simulink model "ISO2631_All_Generation"  (Simulink 7.6)
settings: Solver=ode45  StartTime=0.0  StopTime=1  RelTol=1e-3
settings Model: Creator=Kristian  LastModifiedBy=Kristian
settings RTWCC: GenerateReport=on  LaunchReport=on
settings SimEventsCC: propDiagAttribOutput=1  propDiagFcnCallOutput=1  propDiagStatOutput=0

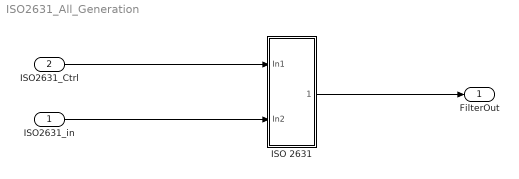
== system ISO2631_All_Generation ==
  ISO2631_in : Inport  OutDataTypeStr=double
  ISO2631_Ctrl : Inport  Port=2  OutDataTypeStr=double
  ISO 2631 : Subsystem
  FilterOut : Outport  OutDataTypeStr=double
  wires:
  ISO2631_Ctrl/1 -> ISO 2631/1(In1)
  ISO 2631/1(Out1) -> FilterOut/1
  ISO2631_in/1 -> ISO 2631/2(In2)

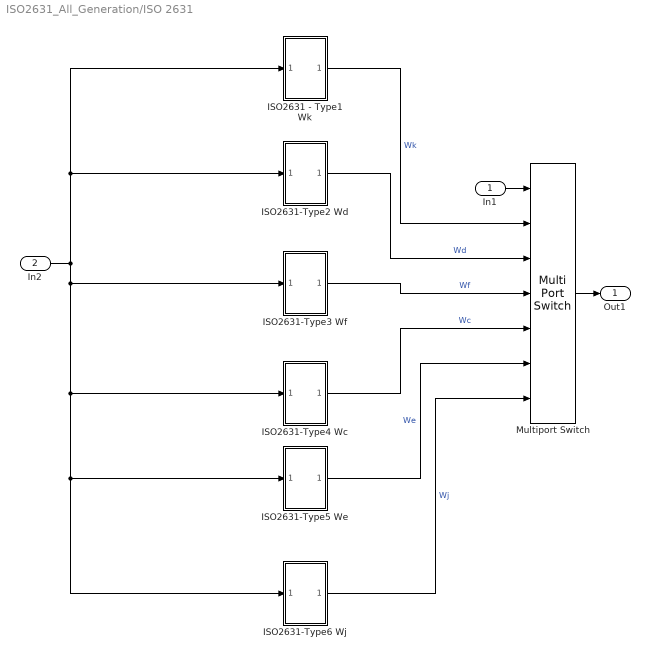
== system ISO2631_All_Generation/ISO 2631 ==
  In1 : Inport
  In2 : Inport  Port=2
  ISO2631 - Type1 Wk : Subsystem
  ISO2631-Type2 Wd : Subsystem
  ISO2631-Type3 Wf : Subsystem
  ISO2631-Type4 Wc : Subsystem
  ISO2631-Type5 We : Subsystem
  ISO2631-Type6 Wj : Subsystem
  Multiport Switch : MultiPortSwitch  DataPortOrder=Specify indices  Inputs=6  DataPortIndices={1,2,3,4,5,6}  zeroidx=off  RndMeth=Ceiling
  Out1 : Outport
  wires:
  In2/1 -> ISO2631 - Type1 Wk/1(In1), ISO2631-Type2 Wd/1(In1), ISO2631-Type3 Wf/1(In1), ISO2631-Type4 Wc/1(In1), ISO2631-Type6 Wj/1(In1), ISO2631-Type5 We/1(In1)
  ISO2631 - Type1 Wk/1(Out1) -> Multiport Switch/2  "Wk"
  ISO2631-Type2 Wd/1(Out1) -> Multiport Switch/3  "Wd"
  ISO2631-Type3 Wf/1(Out1) -> Multiport Switch/4  "Wf"
  ISO2631-Type4 Wc/1(Out1) -> Multiport Switch/5  "Wc"
  ISO2631-Type5 We/1(Out1) -> Multiport Switch/6  "We"
  ISO2631-Type6 Wj/1(Out1) -> Multiport Switch/7  "Wj"
  In1/1 -> Multiport Switch/1
  Multiport Switch/1 -> Out1/1

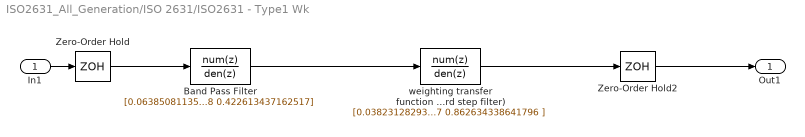
== system ISO2631_All_Generation/ISO 2631/ISO2631 - Type1 Wk ==
  In1 : Inport
  Band Pass Filter : DiscreteFilter  Numerator=|  Denominator=[1.0 -3.16470636644551 3.75293919582273 -2.01084465327318 0.422613437162517]  SampleTime=1/1000
      | [0.0638508113542868 1.33226762955019E-15 -0.127701622708578 4.2188474935756E-15 0.0638508113542855
      | ]
  Zero-Order Hold : ZeroOrderHold  SampleTime=1/1000
  Zero-Order Hold2 : ZeroOrderHold  SampleTime=1/1000
  weighting transfer function (Acceleration-velocity transition + Upward step filter) : DiscreteFilter  Numerator=|  Denominator=|  SampleTime=1/1000
      Numerator=|
      | [0.0382312829345277 -0.0729444373075823 -0.0034621921267961 0.0729450727468253 -0.0347684553684901
      | ]
      Denominator=|
      | [1.0 -3.85371908982878 5.57025894073329 -3.57917165034607 0.862634338641796
      | ]
  Out1 : Outport
  wires:
  Band Pass Filter/1 -> weighting transfer function (Acceleration-velocity transition + Upward step filter)/1
  Zero-Order Hold/1 -> Band Pass Filter/1
  In1/1 -> Zero-Order Hold/1
  weighting transfer function (Acceleration-velocity transition + Upward step filter)/1 -> Zero-Order Hold2/1
  Zero-Order Hold2/1 -> Out1/1

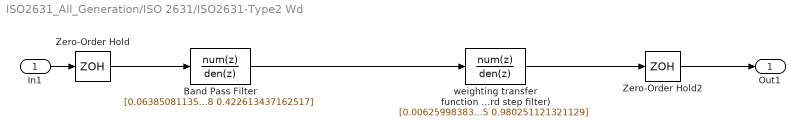
== system ISO2631_All_Generation/ISO 2631/ISO2631-Type2 Wd ==
  In1 : Inport
  Band Pass Filter : DiscreteFilter  Numerator=[0.0638508113542868 1.33226762955019e-15 -0.127701622708578 4.21884749357560e-15 0.0638508113542855]  Denominator=[1 -3.16470636644551 3.75293919582273 -2.01084465327318 0.422613437162517]  SampleTime=1/1000
  Zero-Order Hold : ZeroOrderHold  SampleTime=1/1000
  Zero-Order Hold2 : ZeroOrderHold  SampleTime=1/1000
  weighting transfer function (Acceleration-velocity transition + Upward step filter) : DiscreteFilter  Numerator=[0.00625998383111404 7.81740945390297e-05 -0.00618180973657412]  Denominator=[1 -1.98009477313205 0.980251121321129]  SampleTime=1/1000
  Out1 : Outport
  wires:
  Band Pass Filter/1 -> weighting transfer function (Acceleration-velocity transition + Upward step filter)/1
  Zero-Order Hold/1 -> Band Pass Filter/1
  In1/1 -> Zero-Order Hold/1
  weighting transfer function (Acceleration-velocity transition + Upward step filter)/1 -> Zero-Order Hold2/1
  Zero-Order Hold2/1 -> Out1/1

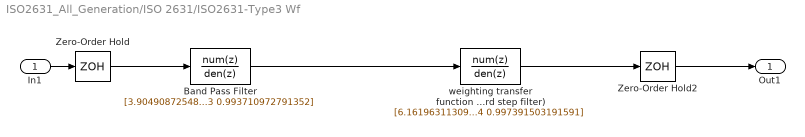
== system ISO2631_All_Generation/ISO 2631/ISO2631-Type3 Wf ==
  In1 : Inport
  Band Pass Filter : DiscreteFilter  Numerator=[3.90490872548277e-06 1.33226762955019e-15 -7.80981745673870e-06 6.66133814775094e-15 3.90490872359539e-06]  Denominator=[1 -3.99369112814028 5.98109324158920 -3.98111308623633 0.993710972791352]  SampleTime=1/1000
  Zero-Order Hold : ZeroOrderHold  SampleTime=1/1000
  Zero-Order Hold2 : ZeroOrderHold  SampleTime=1/1000
  weighting transfer function (Acceleration-velocity transition + Upward step filter) : DiscreteFilter  Numerator=[6.16196311309381e-07 3.02496694359888e-10 -1.23209003710656e-06 -3.02301739196764e-10 6.15893909761134e-07]  Denominator=[1 -3.99738721075116 5.99216592735038 -3.99217021978984 0.997391503191591]  SampleTime=1/1000
  Out1 : Outport
  wires:
  Band Pass Filter/1 -> weighting transfer function (Acceleration-velocity transition + Upward step filter)/1
  Zero-Order Hold/1 -> Band Pass Filter/1
  In1/1 -> Zero-Order Hold/1
  weighting transfer function (Acceleration-velocity transition + Upward step filter)/1 -> Zero-Order Hold2/1
  Zero-Order Hold2/1 -> Out1/1

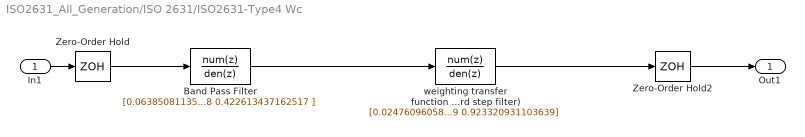
== system ISO2631_All_Generation/ISO 2631/ISO2631-Type4 Wc ==
  In1 : Inport
  Band Pass Filter : DiscreteFilter  Numerator=[0.0638508113542868 1.33226762955019e-15 -0.127701622708578 4.21884749357560e-15 0.0638508113542855]  Denominator=|  SampleTime=1/1000
      | [1 -3.16470636644551 3.75293919582273 -2.01084465327318 0.422613437162517
      | ]
  Zero-Order Hold : ZeroOrderHold  SampleTime=1/1000
  Zero-Order Hold2 : ZeroOrderHold  SampleTime=1/1000
  weighting transfer function (Acceleration-velocity transition + Upward step filter) : DiscreteFilter  Numerator=[0.0247609605891664 0.00121410777362563 -0.0235468528155406]  Denominator=[1 -1.92089271555639 0.923320931103639]  SampleTime=1/1000
  Out1 : Outport
  wires:
  Band Pass Filter/1 -> weighting transfer function (Acceleration-velocity transition + Upward step filter)/1
  Zero-Order Hold/1 -> Band Pass Filter/1
  In1/1 -> Zero-Order Hold/1
  weighting transfer function (Acceleration-velocity transition + Upward step filter)/1 -> Zero-Order Hold2/1
  Zero-Order Hold2/1 -> Out1/1

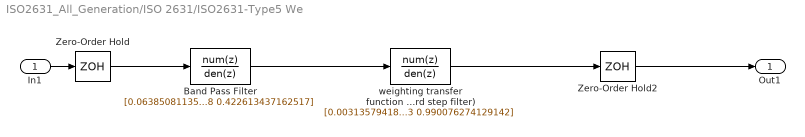
== system ISO2631_All_Generation/ISO 2631/ISO2631-Type5 We ==
  In1 : Inport
  Band Pass Filter : DiscreteFilter  Numerator=[0.0638508113542868 1.33226762955019e-15 -0.127701622708578 4.21884749357560e-15 0.0638508113542855]  Denominator=[1 -3.16470636644551 3.75293919582273 -2.01084465327318 0.422613437162517]  SampleTime=1/1000
  Zero-Order Hold : ZeroOrderHold  SampleTime=1/1000
  Zero-Order Hold2 : ZeroOrderHold  SampleTime=1/1000
  weighting transfer function (Acceleration-velocity transition + Upward step filter) : DiscreteFilter  Numerator=[0.00313579418517251 1.96410717046014e-05 -0.00311615311346891]  Denominator=[1 -1.99003699198573 0.990076274129142]  SampleTime=1/1000
  Out1 : Outport
  wires:
  Band Pass Filter/1 -> weighting transfer function (Acceleration-velocity transition + Upward step filter)/1
  Zero-Order Hold/1 -> Band Pass Filter/1
  In1/1 -> Zero-Order Hold/1
  weighting transfer function (Acceleration-velocity transition + Upward step filter)/1 -> Zero-Order Hold2/1
  Zero-Order Hold2/1 -> Out1/1

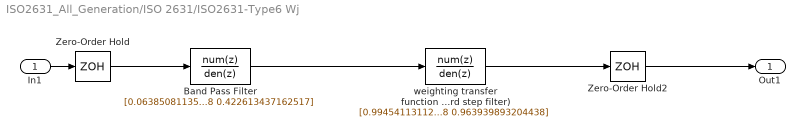
== system ISO2631_All_Generation/ISO 2631/ISO2631-Type6 Wj ==
  In1 : Inport
  Band Pass Filter : DiscreteFilter  Numerator=[0.0638508113542868 1.33226762955019e-15 -0.127701622708578 4.21884749357560e-15 0.0638508113542855]  Denominator=[1 -3.16470636644551 3.75293919582273 -2.01084465327318 0.422613437162517]  SampleTime=1/1000
  Zero-Order Hold : ZeroOrderHold  SampleTime=1/1000
  Zero-Order Hold2 : ZeroOrderHold  SampleTime=1/1000
  weighting transfer function (Acceleration-velocity transition + Upward step filter) : DiscreteFilter  Numerator=[0.994541131125826 -1.96311895053930 0.969122822764292]  Denominator=[1 -1.96284301122498 0.963939893204438]  SampleTime=1/1000
  Out1 : Outport
  wires:
  Band Pass Filter/1 -> weighting transfer function (Acceleration-velocity transition + Upward step filter)/1
  Zero-Order Hold/1 -> Band Pass Filter/1
  In1/1 -> Zero-Order Hold/1
  weighting transfer function (Acceleration-velocity transition + Upward step filter)/1 -> Zero-Order Hold2/1
  Zero-Order Hold2/1 -> Out1/1
